simulink model "sampleModel1822"  (R2023a)
settings: Solver=VariableStepAuto  StartTime=0.0  StopTime=10.0  RelTol=1e-3
libraries: hdlsllib x3, simulink x1
settings Model: Creator=user1  LastModifiedBy=user1

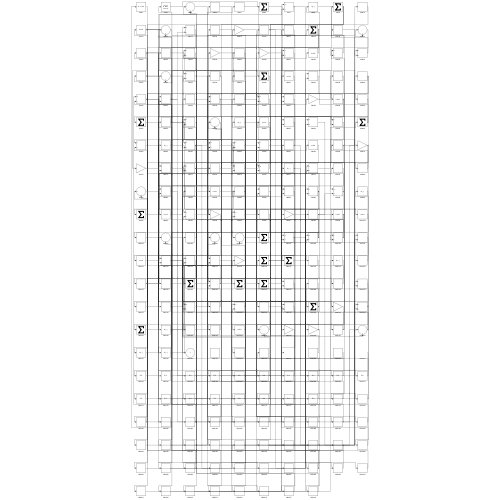
[thumbnail: Simulink's stored preview of the top-level diagram]
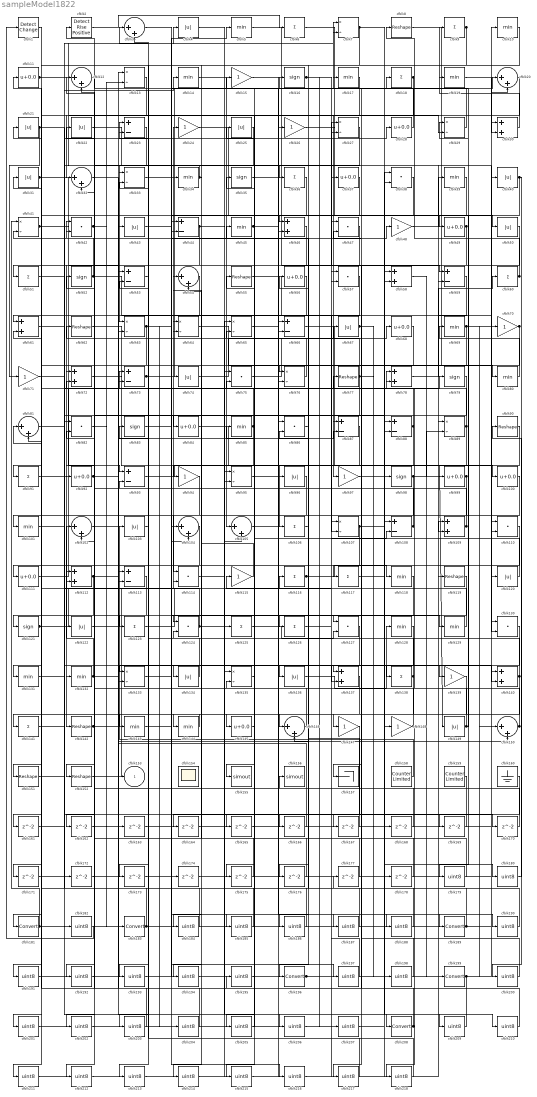
== system sampleModel1822 ==
  cfblk1 : simulink/Logic and Bit Operations/Detect Change  vinit=0  OutDataTypeStr=boolean
      settings: LibrarySourceBlock=|
      | hdlsllib/Logic and Bit
      | Operations/Detect
      | Change
  cfblk{5,10,14,17,19,34,39,45,69,80,85,101,118,128..129,131..132,143..144} (19 alike) : MinMax
  cfblk{11,28,37,49,56,68,84,92,99..100,111,145} (12 alike) : Bias  Bias=0.0  SaturateOnIntegerOverflow=off
  cfblk{3,12,20,32,54,81,102,104..105,146,150} (11 alike) : Sum  Inputs=|++
  cfblk{4,21..22,25,31,40,43,50,67,74,96,103,120,122,134,136,149} (17 alike) : Abs  SaturateOnIntegerOverflow=off
  cfblk{6,9,18,36,51,60,91,106,116..117,123,125..126,138,141} (15 alike) : Sum  Inputs=+
  cfblk{7,13,27,29,33,41,63..65,76,89,95,107,133,135} (15 alike) : Product  Inputs=*/  RndMeth=Zero  SaturateOnIntegerOverflow=on
  cfblk{23,44,53,59,66,73,87..88,93,108,113} (11 alike) : Sum  Inputs=+-
  cfblk{30,46,58,61,72,78,109,112,137,140} (10 alike) : Sum
  cfblk{38,42,47,57,75,82,86,110,114,124,127,130} (12 alike) : DotProduct  OutDataTypeStr=Inherit: Inherit via internal rule
  cfblk{15,24,26,48,70..71,94,97,115,139,147..148} (12 alike) : Gain
  cfblk{8,55,62,77,90,119,142,151..152} (9 alike) : Reshape
  cfblk{16,35,52,79,83,98,121} (7 alike) : Signum
  cfblk154 : Scope
      settings: Floating=on
  cfblk155 : ToWorkspace  VariableName=simout  SaveFormat=Timeseries  SampleTime=-1
  cfblk156 : ToWorkspace  VariableName=simout  SaveFormat=Timeseries  SampleTime=-1
  cfblk157 : Terminator
  cfblk158 : hdlsllib/Sources/Counter Limited  uplimit=7  tsamp=-1
  cfblk159 : hdlsllib/Sources/Counter Limited  uplimit=7  tsamp=-1
  cfblk160 : Ground
  cfblk{161..178} (18 alike) : Delay  SampleTime=1
  cfblk{179..180,182,184..188,190..195,197..198,200..207,209..218} (34 alike) : DataTypeConversion  OutDataTypeStr=uint8  SaturateOnIntegerOverflow=off  RndMeth=Floor
  cfblk{181,183,189,196,199,208} (6 alike) : DataTypeConversion  SaturateOnIntegerOverflow=off  RndMeth=Floor
  cfblk2 : hdlsllib/Logic and Bit Operations/Detect Rise Positive  vinit=0  OutDataTypeStr=boolean
  cfblk153 : Outport  VectorParamsAs1DForOutWhenUnconnected=off
  wires:
  cfblk111/1 -> cfblk79/1
  cfblk31/1 -> cfblk93/1, cfblk36/1
  cfblk11/1 -> cfblk63/1, cfblk29/2, cfblk7/2
  cfblk8/1 -> cfblk146/1
  cfblk98/1 -> cfblk149/1, cfblk89/2, cfblk122/1
  cfblk14/1 -> cfblk105/1
  cfblk158/1 -> cfblk103/1
  cfblk24/1 -> cfblk50/1
  cfblk44/1 -> cfblk142/1, cfblk210/1
  cfblk159/1 -> cfblk156/1
  cfblk57/1 -> cfblk132/1
  cfblk140/1 -> cfblk145/1, cfblk115/1
  cfblk116/1 -> cfblk118/1, cfblk78/1
  cfblk5/1 -> cfblk59/1
  cfblk64/1 -> cfblk80/1
  cfblk73/1 -> cfblk20/1, cfblk166/1, cfblk203/1
  cfblk82/1 -> cfblk183/1
  cfblk127/1 -> cfblk136/1
  cfblk84/1 -> cfblk100/1
  cfblk136/1 -> cfblk128/1
  cfblk139/1 -> cfblk147/1
  cfblk72/1 -> cfblk125/1
  cfblk89/1 -> cfblk157/1, cfblk54/2
  cfblk120/1 -> cfblk85/1
  cfblk148/1 -> cfblk113/1, cfblk218/1
  cfblk78/1 -> cfblk60/1
  cfblk107/1 -> cfblk180/1, cfblk201/1
  cfblk56/1 -> cfblk61/1
  cfblk129/1 -> cfblk25/1
  cfblk152/1 -> cfblk66/2
  cfblk55/1 -> cfblk120/1
  cfblk20/1 -> cfblk155/1
  cfblk85/1 -> cfblk24/1, cfblk214/1
  cfblk19/1 -> cfblk30/2
  cfblk142/1 -> cfblk64/1, cfblk114/2
  cfblk99/1 -> cfblk93/2, cfblk215/1
  cfblk58/1 -> cfblk199/1
  cfblk117/1 -> cfblk98/1
  cfblk70/1 -> cfblk143/1, cfblk133/1
  cfblk137/1 -> cfblk144/1
  cfblk124/1 -> cfblk127/1, cfblk21/1
  cfblk21/1 -> cfblk71/1, cfblk84/1, cfblk87/1
  cfblk60/1 -> cfblk51/1, cfblk8/1
  cfblk94/1 -> cfblk152/1
  cfblk87/1 -> cfblk106/1
  cfblk96/1 -> cfblk114/1
  cfblk63/1 -> cfblk5/1, cfblk73/2, cfblk204/1
  cfblk132/1 -> cfblk102/1, cfblk87/2
  cfblk18/1 -> cfblk32/1, cfblk32/2
  cfblk144/1 -> cfblk141/1
  cfblk68/1 -> cfblk121/1
  cfblk146/1 -> cfblk22/1
  cfblk2/1 -> cfblk6/1
  cfblk65/1 -> cfblk88/2
  cfblk150/1 -> cfblk29/1, cfblk23/2
  cfblk34/1 -> cfblk33/1, cfblk124/1
  cfblk93/1 -> cfblk96/1
  cfblk29/1 -> cfblk2/1
  cfblk1/1 -> cfblk181/1
  cfblk7/1 -> cfblk193/1, cfblk209/1
  cfblk75/1 -> cfblk68/1
  cfblk62/1 -> cfblk105/2
  cfblk13/1 -> cfblk111/1
  cfblk122/1 -> cfblk95/1
  cfblk138/1 -> cfblk124/2, cfblk167/1
  cfblk17/1 -> cfblk97/1
  cfblk28/1 -> cfblk7/1
  cfblk52/1 -> cfblk107/2, cfblk75/1, cfblk11/1
  cfblk134/1 -> cfblk23/1
  cfblk26/1 -> cfblk49/1
  cfblk123/1 -> cfblk37/1
  cfblk35/1 -> cfblk189/1
  cfblk125/1 -> cfblk127/2
  cfblk47/1 -> cfblk196/1
  cfblk126/1 -> cfblk108/2
  cfblk37/1 -> cfblk131/1
  cfblk91/1 -> cfblk74/1
  cfblk40/1 -> cfblk44/2, cfblk99/1, cfblk200/1
  cfblk102/1 -> cfblk150/2
  cfblk69/1 -> cfblk20/2, cfblk94/1
  cfblk25/1 -> cfblk72/1
  cfblk59/1 -> cfblk109/2
  cfblk103/1 -> cfblk33/2
  cfblk151/1 -> cfblk14/1
  cfblk79/1 -> cfblk112/1
  cfblk101/1 -> cfblk137/1
  cfblk88/1 -> cfblk31/1, cfblk146/2, cfblk175/1
  cfblk77/1 -> cfblk62/1, cfblk133/2, cfblk168/1
  cfblk22/1 -> cfblk130/2
  cfblk76/1 -> cfblk52/1
  cfblk106/1 -> cfblk56/1
  cfblk45/1 -> cfblk15/1, cfblk188/1
  cfblk92/1 -> cfblk43/1, cfblk42/1
  cfblk121/1 -> cfblk34/1, cfblk4/1
  cfblk135/1 -> cfblk45/1
  cfblk66/1 -> cfblk148/1
  cfblk80/1 -> cfblk69/1
  cfblk81/1 -> cfblk208/1
  cfblk16/1 -> cfblk59/2, cfblk207/1
  cfblk131/1 -> cfblk116/1
  cfblk36/1 -> cfblk91/1
  cfblk105/1 -> cfblk139/1
  cfblk9/1 -> cfblk76/1, cfblk126/1, cfblk161/1
  cfblk115/1 -> cfblk54/1
  cfblk30/1 -> cfblk9/1
  cfblk143/1 -> cfblk48/1
  cfblk71/1 -> cfblk28/1
  cfblk145/1 -> cfblk55/1
  cfblk95/1 -> cfblk18/1
  cfblk54/1 -> cfblk92/1
  cfblk6/1 -> cfblk89/1
  cfblk53/1 -> cfblk123/1
  cfblk112/1 -> cfblk151/1, cfblk137/2, cfblk138/1
  cfblk41/1 -> cfblk153/1, cfblk140/2
  cfblk49/1 -> cfblk117/1, cfblk76/2
  cfblk109/1 -> cfblk65/2, cfblk72/2
  cfblk33/1 -> cfblk46/1
  cfblk42/1 -> cfblk13/2, cfblk163/1
  cfblk141/1 -> cfblk73/1
  cfblk67/1 -> cfblk17/1, cfblk198/1
  cfblk43/1 -> cfblk129/1
  cfblk39/1 -> cfblk46/2
  cfblk46/1 -> cfblk63/2
  cfblk48/1 -> cfblk39/1
  cfblk149/1 -> cfblk19/1, cfblk78/2
  cfblk128/1 -> cfblk134/1
  cfblk133/1 -> cfblk16/1
  cfblk74/1 -> cfblk67/1
  cfblk108/1 -> cfblk101/1, cfblk53/2, cfblk83/1
  cfblk23/1 -> cfblk162/1
  cfblk162/1 -> cfblk107/1
  cfblk147/1 -> cfblk164/1
  cfblk164/1 -> cfblk140/1
  cfblk61/1 -> cfblk165/1
  cfblk165/1 -> cfblk66/1
  cfblk166/1 -> cfblk13/1
  cfblk167/1 -> cfblk41/2
  cfblk168/1 -> cfblk112/2
  cfblk114/1 -> cfblk169/1
  cfblk169/1 -> cfblk65/1
  cfblk97/1 -> cfblk170/1
  cfblk170/1 -> cfblk109/1
  cfblk118/1 -> cfblk171/1
  cfblk171/1 -> cfblk44/1
  cfblk51/1 -> cfblk172/1
  cfblk172/1 -> cfblk30/1
  cfblk130/1 -> cfblk173/1
  cfblk83/1 -> cfblk174/1
  cfblk174/1 -> cfblk88/1
  cfblk175/1 -> cfblk42/2
  cfblk100/1 -> cfblk176/1
  cfblk176/1 -> cfblk113/2
  cfblk177/1 -> cfblk75/2
  cfblk178/1 -> cfblk64/2
  cfblk90/1 -> cfblk179/1
  cfblk179/1 -> cfblk57/1
  cfblk180/1 -> cfblk90/1
  cfblk181/1 -> cfblk57/2, cfblk41/1
  cfblk161/1 -> cfblk182/1
  cfblk182/1 -> cfblk1/1
  cfblk183/1 -> cfblk102/2, cfblk40/1
  cfblk50/1 -> cfblk184/1
  cfblk184/1 -> cfblk82/1
  cfblk163/1 -> cfblk185/1
  cfblk185/1 -> cfblk82/2
  cfblk86/1 -> cfblk186/1
  cfblk186/1 -> cfblk61/2
  cfblk15/1 -> cfblk187/1
  cfblk187/1 -> cfblk86/1
  cfblk188/1 -> cfblk86/2
  cfblk189/1 -> cfblk177/1, cfblk70/1
  cfblk4/1 -> cfblk190/1
  cfblk190/1 -> cfblk35/1
  cfblk104/1 -> cfblk191/1
  cfblk191/1 -> cfblk130/1
  cfblk110/1 -> cfblk192/1
  cfblk192/1 -> cfblk104/1
  cfblk193/1 -> cfblk104/2
  cfblk10/1 -> cfblk194/1
  cfblk194/1 -> cfblk110/1
  cfblk195/1 -> cfblk10/1
  cfblk196/1 -> cfblk110/2, cfblk108/1
  cfblk173/1 -> cfblk197/1
  cfblk197/1 -> cfblk47/1
  cfblk198/1 -> cfblk47/2
  cfblk199/1 -> cfblk195/1, cfblk150/1
  cfblk200/1 -> cfblk58/1
  cfblk201/1 -> cfblk58/2
  cfblk12/1 -> cfblk202/1
  cfblk202/1 -> cfblk135/1
  cfblk203/1 -> cfblk12/1
  cfblk204/1 -> cfblk12/2
  cfblk38/1 -> cfblk205/1
  cfblk205/1 -> cfblk135/2
  cfblk32/1 -> cfblk206/1
  cfblk206/1 -> cfblk38/1
  cfblk207/1 -> cfblk38/2
  cfblk208/1 -> cfblk53/1, cfblk77/1
  cfblk209/1 -> cfblk81/1
  cfblk210/1 -> cfblk81/2
  cfblk119/1 -> cfblk211/1
  cfblk211/1 -> cfblk26/1
  cfblk113/1 -> cfblk212/1
  cfblk212/1 -> cfblk119/1
  cfblk27/1 -> cfblk213/1
  cfblk213/1 -> cfblk95/2
  cfblk214/1 -> cfblk27/1
  cfblk215/1 -> cfblk27/2
  cfblk3/1 -> cfblk216/1
  cfblk216/1 -> cfblk178/1
  cfblk160/1 -> cfblk217/1
  cfblk217/1 -> cfblk3/1
  cfblk218/1 -> cfblk3/2
